simulink model "Hinf_BS_Comparison"  (R2026a)
settings: Solver=ode23tb  StopTime=175  FixedStep=0.0001  MaxStep=0.02  RelTol=1e-9  AbsTol=1e-12
PostLoadFcn:
  | init_comparison(bdroot);
InitFcn:
  | init_comparison(bdroot);
model workspace (MAT data in the model file):
  A = [-4.33427458178e-18 -1739.27628419 -1.9879507565e-12 -947.702562069 9.25490783271 -3.87188490855e-14 40.5994463199 -1.82279284791e-15 1.34368571874e-07 -8.90717137351e-10 -711.607566004 -711.607566004 ... (196 elements, 14x14)]
  B = [-1.75563782385e-19 2.23785567073e-19 -10165.2431057 -49.2726170531 5.13589910552 -5.90943945895 6.81435391425 45.4160051294 1073741824 17236611.4468 7.60467680903e-16 -1.03174259462e-14 ... (14 elements, 14x1)]
  C = [-313107.329042 -2686499.93691 37750.0108104 101565.096764 -37.2177294622 -2820.69827595 3048.09156473 3382.76066655 -2.10142044744 -107.98720369 -2843187.08558 -2796371.67099 ... (14 elements, 1x14)]
  D = 0
  a1 = 3
  a2 = 3
  a3 = 3
  a4 = 3
  b = -100
  k1 = 9.81
  k1_0 = 9.81
  k1_3 = 7.3575
  k2 = 0.555555555556
  k2_0 = 1.11111111111
  k2_3 = 6.66666666667
  k3 = 2.9
  k3_0 = 2
  k3_3 = 7.93333333333
  k4 = 1.8
  k4_0 = 0.9
  k4_3 = 0.45
  k5 = 0.620689655172
  k5_0 = 0.45
  k5_3 = 0.0567226890756
  r_test = [0 0.02 0.04 0.06 0.08 0.1 0.12 0.14 0.16 0.18 0.2 0.22 ... (17570 elements, 8785x2)]
  w = 500
(part 2 of 2)

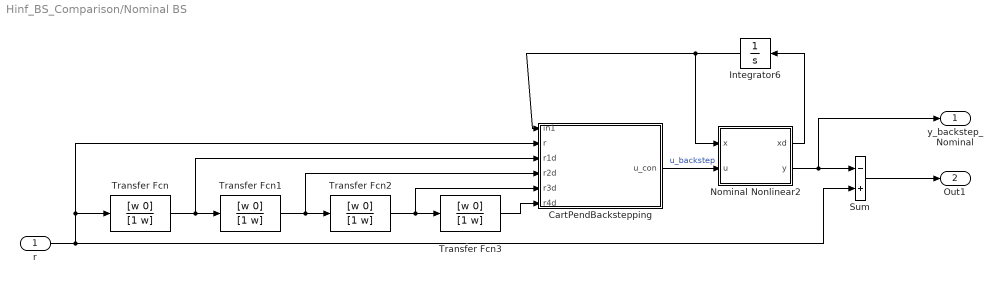
== system Hinf_BS_Comparison/Nominal BS ==
  r : Inport
  CartPendBackstepping : MATLAB Function  TreatAsAtomicUnit=on
  Integrator6 : Integrator  InitialCondition=zeros(4, 1)
  Nominal Nonlinear2 : MATLAB Function  TreatAsAtomicUnit=on
  Sum : Sum  Inputs=-+
  Transfer Fcn{,1..3} (4 alike) : TransferFcn  Numerator=[w 0]  Denominator=[1 w]
  y_backstep_Nominal : Outport
  Out1 : Outport  Port=2
  wires:
  Sum/1 -> Out1/1
  Nominal Nonlinear2/2(y) -> y_backstep_Nominal/1, Sum/1
  Transfer Fcn3/1 -> CartPendBackstepping/6(r4d)
  Transfer Fcn1/1 -> Transfer Fcn2/1, CartPendBackstepping/4(r2d)
  Nominal Nonlinear2/1(xd) -> Integrator6/1
  Transfer Fcn/1 -> Transfer Fcn1/1, CartPendBackstepping/3(r1d)
  Transfer Fcn2/1 -> Transfer Fcn3/1, CartPendBackstepping/5(r3d)
  Integrator6/1 -> CartPendBackstepping/1(in1), Nominal Nonlinear2/1(x)
  CartPendBackstepping/1(u_con) -> Nominal Nonlinear2/2(u)  "u_backstep"
  r/1 -> CartPendBackstepping/2(r), Transfer Fcn/1, Sum/2

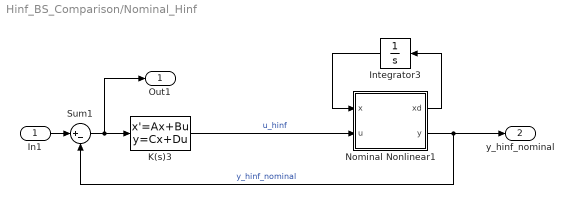
== system Hinf_BS_Comparison/Nominal_Hinf ==
  In1 : Inport
  Integrator3 : Integrator  InitialCondition=zeros(4, 1)
  K(s)3 : StateSpace  A=A  B=B  C=C  D=D  InitialCondition=0
  Nominal Nonlinear1 : MATLAB Function  TreatAsAtomicUnit=on
  Sum1 : Sum  Inputs=|+-
  Out1 : Outport
  y_hinf_nominal : Outport  Port=2
  wires:
  In1/1 -> Sum1/1
  Integrator3/1 -> Nominal Nonlinear1/1(x)
  Nominal Nonlinear1/2(y) -> y_hinf_nominal/1, Sum1/2  "y_hinf_nominal"
  K(s)3/1 -> Nominal Nonlinear1/2(u)  "u_hinf"
  Nominal Nonlinear1/1(xd) -> Integrator3/1
  Sum1/1 -> Out1/1, K(s)3/1

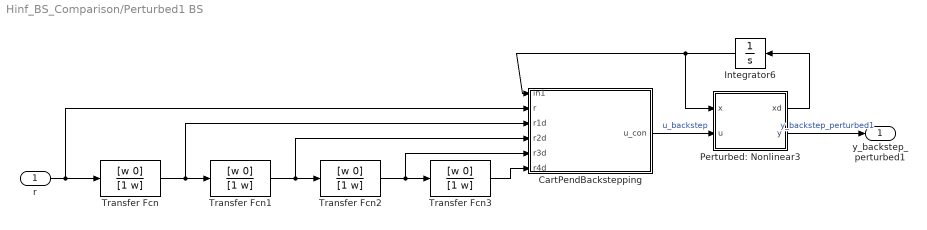
== system Hinf_BS_Comparison/Perturbed1 BS ==
  r : Inport
  CartPendBackstepping : MATLAB Function  TreatAsAtomicUnit=on
  Integrator6 : Integrator  InitialCondition=zeros(4, 1)
  Perturbed: Nonlinear3 : MATLAB Function  TreatAsAtomicUnit=on
  Transfer Fcn{,1..3} (4 alike) : TransferFcn  Numerator=[w 0]  Denominator=[1 w]
  y_backstep_perturbed1 : Outport
  wires:
  Integrator6/1 -> CartPendBackstepping/1(in1), Perturbed: Nonlinear3/1(x)
  Transfer Fcn3/1 -> CartPendBackstepping/6(r4d)
  Transfer Fcn2/1 -> Transfer Fcn3/1, CartPendBackstepping/5(r3d)
  Perturbed: Nonlinear3/1(xd) -> Integrator6/1
  CartPendBackstepping/1(u_con) -> Perturbed: Nonlinear3/2(u)  "u_backstep"
  Transfer Fcn/1 -> Transfer Fcn1/1, CartPendBackstepping/3(r1d)
  Transfer Fcn1/1 -> Transfer Fcn2/1, CartPendBackstepping/4(r2d)
  Perturbed: Nonlinear3/2(y) -> y_backstep_perturbed1/1  "y_backstep_perturbed1"
  r/1 -> CartPendBackstepping/2(r), Transfer Fcn/1

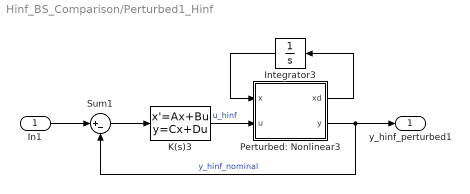
== system Hinf_BS_Comparison/Perturbed1_Hinf ==
  In1 : Inport
  Integrator3 : Integrator  InitialCondition=zeros(4, 1)
  K(s)3 : StateSpace  A=A  B=B  C=C  D=D  InitialCondition=0
  Perturbed: Nonlinear3 : MATLAB Function  TreatAsAtomicUnit=on
  Sum1 : Sum  Inputs=|+-
  y_hinf_perturbed1 : Outport
  wires:
  Integrator3/1 -> Perturbed: Nonlinear3/1(x)
  Perturbed: Nonlinear3/2(y) -> y_hinf_perturbed1/1, Sum1/2  "y_hinf_nominal"
  K(s)3/1 -> Perturbed: Nonlinear3/2(u)  "u_hinf"
  Perturbed: Nonlinear3/1(xd) -> Integrator3/1
  Sum1/1 -> K(s)3/1
  In1/1 -> Sum1/1

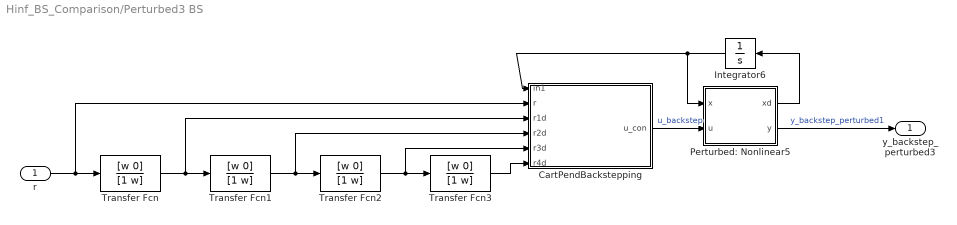
== system Hinf_BS_Comparison/Perturbed3 BS ==
  r : Inport
  CartPendBackstepping : MATLAB Function  TreatAsAtomicUnit=on
  Integrator6 : Integrator  InitialCondition=zeros(4, 1)
  Perturbed: Nonlinear5 : MATLAB Function  TreatAsAtomicUnit=on
  Transfer Fcn{,1..3} (4 alike) : TransferFcn  Numerator=[w 0]  Denominator=[1 w]
  y_backstep_perturbed3 : Outport
  wires:
  Integrator6/1 -> Perturbed: Nonlinear5/1(x), CartPendBackstepping/1(in1)
  Transfer Fcn3/1 -> CartPendBackstepping/6(r4d)
  Transfer Fcn2/1 -> Transfer Fcn3/1, CartPendBackstepping/5(r3d)
  Perturbed: Nonlinear5/1(xd) -> Integrator6/1
  CartPendBackstepping/1(u_con) -> Perturbed: Nonlinear5/2(u)  "u_backstep"
  Transfer Fcn/1 -> Transfer Fcn1/1, CartPendBackstepping/3(r1d)
  Transfer Fcn1/1 -> Transfer Fcn2/1, CartPendBackstepping/4(r2d)
  Perturbed: Nonlinear5/2(y) -> y_backstep_perturbed3/1  "y_backstep_perturbed1"
  r/1 -> Transfer Fcn/1, CartPendBackstepping/2(r)

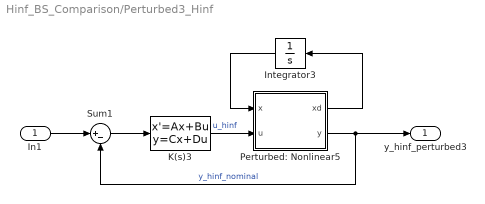
== system Hinf_BS_Comparison/Perturbed3_Hinf ==
  In1 : Inport
  Integrator3 : Integrator  InitialCondition=zeros(4, 1)
  K(s)3 : StateSpace  A=A  B=B  C=C  D=D  InitialCondition=0
  Perturbed: Nonlinear5 : MATLAB Function  TreatAsAtomicUnit=on
  Sum1 : Sum  Inputs=|+-
  y_hinf_perturbed3 : Outport
  wires:
  Integrator3/1 -> Perturbed: Nonlinear5/1(x)
  Perturbed: Nonlinear5/2(y) -> y_hinf_perturbed3/1, Sum1/2  "y_hinf_nominal"
  K(s)3/1 -> Perturbed: Nonlinear5/2(u)  "u_hinf"
  Perturbed: Nonlinear5/1(xd) -> Integrator3/1
  Sum1/1 -> K(s)3/1
  In1/1 -> Sum1/1

== matlab function Hinf_BS_Comparison/Perturbed3_Hinf/Perturbed: Nonlinear5 ==
  data: x input; u input; xd output; k1_3 parameter; k2_3 parameter; k3_3 parameter; k4_3 parameter; k5_3 parameter; b parameter; y output
function [xd, y] = cart_pend(x, u, k1_3, k2_3, k3_3, k4_3, k5_3, b)
xd = [x(2);
      -b^2*x(1) + 2*b*x(2) + b^2*u;
      x(4);
      (-k1_3*sin(x(3)) - k2_3*x(4) - cos(x(3))/k3_3 .* (x(1) + k4_3*sin(x(3)).*x(4).^2))./(1 - k5_3*cos(x(3)).^2)];
y = x(3);

== matlab function Hinf_BS_Comparison/Perturbed3 BS/CartPendBackstepping ==
  data: in1 input; u_con output; r input; r1d input; r2d input; r3d input; r4d input; a1 parameter; a2 parameter; a3 parameter; a4 parameter
function u_con = CartPendBackstepping(in1,r,r1d,r2d,r3d,r4d,a1, a2, a3, a4)
%#codegen


p1 = in1(1,:);
p2 = in1(2,:);
x1 = in1(3,:);
x2 = in1(4,:);
t2 = cos(x1);
t3 = sin(x1);
t4 = a1.*a2;
t5 = x1.*2.0;
t6 = x2.^2;
t7 = x2.^3;
t16 = -x1;
t17 = -x2;
t24 = x2.*(1.0e+1./9.0);
t8 = cos(t5);
t9 = t2.^2;
t10 = t2.^3;
t12 = t2.^5;
t14 = sin(t5);
t15 = t3.^3;
t18 = p1.*t3.*5.0e+1;
t19 = t2.*9.81e+2;
t22 = (p1.*t2)./2.0;
t28 = t3.*(9.81e+2./1.0e+2);
t34 = t2.*t3.*t6.*(9.0./2.0e+1);
t11 = t9.^2;
t13 = t9.^3;
t20 = t8.*9.0;
t21 = t9.*9.0;
t23 = -t18;
t25 = t8.*8.1e+1;
t26 = t14.*x2.*1.62e+2;
t27 = t8.*(9.0./2.0);
t32 = t6.*t14.*(9.0./4.0e+1);
t42 = t22+t24+t28+t34;
t29 = t20-3.1e+1;
t30 = t21-2.0e+1;
t31 = t26+4.0e+2;
t33 = t25-2.79e+2;
t37 = t27-3.1e+1./2.0;
t43 = t22+t24+t28+t32;
t35 = 1.0./t30;
t38 = 1.0./t33;
t39 = 1.0./t37;
t36 = t35.^2;
t40 = t31.*t38;
t41 = a1+a2+t40;
et1 = a1.*3.6e+5+a3.*3.6e+5-t2.*3.1392e+6-t6.*9.0e+5+t10.*5.2974e+6-a1.*t2.*3.5316e+5-a2.*t2.*3.5316e+5-a3.*t2.*3.5316e+5+a1.*t6.*1.62e+5+a3.*t4.*3.6e+5+a2.*t6.*1.62e+5+a3.*t6.*1.62e+5-a1.*t9.*4.86e+5-a1.*t10.*1.430298e+6+a1.*t11.*2.187e+5-a2.*t10.*1.430298e+6-a3.*t9.*4.86e+5+a1.*t12.*7.15149e+5-a3.*t10.*1.430298e+6-a1.*t13.*3.2805e+4;
et2 = a2.*t12.*7.15149e+5+a3.*t11.*2.187e+5+a3.*t12.*7.15149e+5-a3.*t13.*3.2805e+4-p1.*t3.*4.7e+5+p2.*t3.*1.8e+5+p1.*t15.*2.7e+5+t6.*t9.*5.85e+5+t6.*t11.*8.1e+5-t7.*t14.*4.05e+4+t3.*x2.*7.663572e+6-t14.*x2.*4.0e+5-t15.*x2.*1.0488852e+7+a1.*p1.*t3.*1.8e+5+a2.*p1.*t3.*1.8e+5+a3.*p1.*t3.*1.8e+5-a1.*t6.*t9.*3.24e+5-a3.*t4.*t9.*4.86e+5-a2.*t6.*t9.*3.24e+5+a1.*t6.*t11.*1.12995e+5;
et3 = a3.*t4.*t11.*2.187e+5-a3.*t6.*t9.*3.24e+5+a2.*t6.*t11.*1.12995e+5-a3.*t4.*t13.*3.2805e+4+a3.*t6.*t11.*1.12995e+5+a1.*t14.*x2.*1.8e+5+a2.*t14.*x2.*1.8e+5+a3.*t14.*x2.*1.8e+5-p2.*t3.*t11.*3.645e+4-p1.*t2.*x2.*6.3e+5+p1.*t10.*x2.*7.533e+5+p1.*t12.*x2.*1.0935e+5+t3.*t7.*t10.*6.7797e+5+t3.*t11.*x2.*2.145447e+6-a1.*p1.*t3.*t11.*3.645e+4-a2.*p1.*t3.*t11.*3.645e+4-a3.*p1.*t3.*t11.*3.645e+4-a1.*t3.*t10.*x2.*1.62e+5;
et4 = a2.*t3.*t10.*x2.*-1.62e+5-a3.*t3.*t10.*x2.*1.62e+5;
et5 = r4d+r1d.*(a1+a3+a3.*t4)+r3d.*(a1+a2+a3)+a4.*(r1d+r3d+t17+a1.*(r+t16)+t17.*(t4+(t19+t23+t6.*t8.*4.5e+1)./(t8.*(4.5e+1./2.0)-1.55e+2./2.0)+t14.*t39.^2.*t43.*1.8e+2+1.0)+r1d.*(t4+1.0)+a3.*(r+r2d+t16+a1.*r1d+a1.*t17+a2.*(r1d+t17+a1.*r+a1.*t16)-(t3.*8.829e+3+x2.*1.0e+3+p1.*t2.*4.5e+2+t6.*t14.*(4.05e+2./2.0))./(t8.*(4.05e+2./2.0)-6.975e+2))+r2d.*(a1+a2)-p2.*t2.*t39.*1.0e+1-t39.*t41.*t43.*2.0e+1)+r2d.*(t4+a1.*a3+a2.*a3+2.0)+t2.*t35.*(p1.*1.0e+5+p2.*2.0e+3);
et6 = (t35.^3.*x2.*(et1+et2+et3+et4))./4.5e+1-t35.*t42.*(t4+a3.*t41-(t6.*4.5e+1+t18-t19-t6.*t9.*9.0e+1)./(t9.*4.5e+1-1.0e+2)+1.0./t29.^2.*x2.*(t14.*8.0e+2+x2.*3.24e+2-t8.*x2.*1.116e+3)+(t41.*(t14.*x2.*(9.0./2.0e+1)+1.0e+1./9.0).*4.0e+1)./t29+t2.*t3.*t36.*t42.*7.2e+2+2.0).*2.0e+1-p2.*t36.*(t2.*2.0e+2-a1.*t2.*1.8e+2-a2.*t2.*1.8e+2-a3.*t2.*1.8e+2+a1.*t10.*8.1e+1+a2.*t10.*8.1e+1+a3.*t10.*8.1e+1+t3.*x2.*1.8e+2+t3.*t9.*x2.*2.43e+2).*(1.0e+1./9.0);
u_con = ((et5+et6).*(t9.*(9.0./2.0e+1)-1.0))./(t2.*5.0e+3);

% Complete the final recursion: dot(z3) = -a4*z3 - z2.
a_nom = (-9.81*sin(x1)-x2/0.9-0.5*p1*cos(x1) ...
    -0.45*cos(x1)*sin(x1)*x2.^2)./(1-0.45*cos(x1).^2);
b_nom = -0.5*cos(x1)./(1-0.45*cos(x1).^2);
z2 = r2d-a_nom+(a1+a2).*(r1d-x2)+(a1.*a2+1).*(r-x1);
u_con = u_con + z2./(1.0e4*b_nom);
end

== matlab function Hinf_BS_Comparison/Perturbed3 BS/Perturbed: Nonlinear5 ==
  data: x input; u input; xd output; k1_3 parameter; k2_3 parameter; k3_3 parameter; k4_3 parameter; k5_3 parameter; b parameter; y output
function [xd, y] = cart_pend(x, u, k1_3, k2_3, k3_3, k4_3, k5_3, b)
xd = [x(2);
      -b^2*x(1) + 2*b*x(2) + b^2*u;
      x(4);
      (-k1_3*sin(x(3)) - k2_3*x(4) - cos(x(3))/k3_3 .* (x(1) + k4_3*sin(x(3)).*x(4).^2))./(1 - k5_3*cos(x(3)).^2)];
y = x(3);

== matlab function Hinf_BS_Comparison/Nominal_Hinf/Nominal Nonlinear1 ==
  data: x input; u input; xd output; k1_0 parameter; k2_0 parameter; k3_0 parameter; k4_0 parameter; k5_0 parameter; b parameter; y output
function [xd, y] = cart_pend(x, u, k1_0, k2_0, k3_0, k4_0, k5_0, b)

xd = [x(2);
      -b^2*x(1) + 2*b*x(2) + b^2*u;
      x(4);
      (-k1_0*sin(x(3)) - k2_0*x(4) - cos(x(3))/k3_0 .* (x(1) + k4_0*sin(x(3)).*x(4).^2))./(1 - k5_0*cos(x(3)).^2)];

y = x(3);

== matlab function Hinf_BS_Comparison/Nominal BS/CartPendBackstepping ==
  data: in1 input; u_con output; r input; r1d input; r2d input; r3d input; r4d input; a1 parameter; a2 parameter; a3 parameter; a4 parameter
function u_con = CartPendBackstepping(in1,r,r1d,r2d,r3d,r4d,a1, a2, a3, a4)
%#codegen


p1 = in1(1,:);
p2 = in1(2,:);
x1 = in1(3,:);
x2 = in1(4,:);
t2 = cos(x1);
t3 = sin(x1);
t4 = a1.*a2;
t5 = x1.*2.0;
t6 = x2.^2;
t7 = x2.^3;
t16 = -x1;
t17 = -x2;
t24 = x2.*(1.0e+1./9.0);
t8 = cos(t5);
t9 = t2.^2;
t10 = t2.^3;
t12 = t2.^5;
t14 = sin(t5);
t15 = t3.^3;
t18 = p1.*t3.*5.0e+1;
t19 = t2.*9.81e+2;
t22 = (p1.*t2)./2.0;
t28 = t3.*(9.81e+2./1.0e+2);
t34 = t2.*t3.*t6.*(9.0./2.0e+1);
t11 = t9.^2;
t13 = t9.^3;
t20 = t8.*9.0;
t21 = t9.*9.0;
t23 = -t18;
t25 = t8.*8.1e+1;
t26 = t14.*x2.*1.62e+2;
t27 = t8.*(9.0./2.0);
t32 = t6.*t14.*(9.0./4.0e+1);
t42 = t22+t24+t28+t34;
t29 = t20-3.1e+1;
t30 = t21-2.0e+1;
t31 = t26+4.0e+2;
t33 = t25-2.79e+2;
t37 = t27-3.1e+1./2.0;
t43 = t22+t24+t28+t32;
t35 = 1.0./t30;
t38 = 1.0./t33;
t39 = 1.0./t37;
t36 = t35.^2;
t40 = t31.*t38;
t41 = a1+a2+t40;
et1 = a1.*3.6e+5+a3.*3.6e+5-t2.*3.1392e+6-t6.*9.0e+5+t10.*5.2974e+6-a1.*t2.*3.5316e+5-a2.*t2.*3.5316e+5-a3.*t2.*3.5316e+5+a1.*t6.*1.62e+5+a3.*t4.*3.6e+5+a2.*t6.*1.62e+5+a3.*t6.*1.62e+5-a1.*t9.*4.86e+5-a1.*t10.*1.430298e+6+a1.*t11.*2.187e+5-a2.*t10.*1.430298e+6-a3.*t9.*4.86e+5+a1.*t12.*7.15149e+5-a3.*t10.*1.430298e+6-a1.*t13.*3.2805e+4;
et2 = a2.*t12.*7.15149e+5+a3.*t11.*2.187e+5+a3.*t12.*7.15149e+5-a3.*t13.*3.2805e+4-p1.*t3.*4.7e+5+p2.*t3.*1.8e+5+p1.*t15.*2.7e+5+t6.*t9.*5.85e+5+t6.*t11.*8.1e+5-t7.*t14.*4.05e+4+t3.*x2.*7.663572e+6-t14.*x2.*4.0e+5-t15.*x2.*1.0488852e+7+a1.*p1.*t3.*1.8e+5+a2.*p1.*t3.*1.8e+5+a3.*p1.*t3.*1.8e+5-a1.*t6.*t9.*3.24e+5-a3.*t4.*t9.*4.86e+5-a2.*t6.*t9.*3.24e+5+a1.*t6.*t11.*1.12995e+5;
et3 = a3.*t4.*t11.*2.187e+5-a3.*t6.*t9.*3.24e+5+a2.*t6.*t11.*1.12995e+5-a3.*t4.*t13.*3.2805e+4+a3.*t6.*t11.*1.12995e+5+a1.*t14.*x2.*1.8e+5+a2.*t14.*x2.*1.8e+5+a3.*t14.*x2.*1.8e+5-p2.*t3.*t11.*3.645e+4-p1.*t2.*x2.*6.3e+5+p1.*t10.*x2.*7.533e+5+p1.*t12.*x2.*1.0935e+5+t3.*t7.*t10.*6.7797e+5+t3.*t11.*x2.*2.145447e+6-a1.*p1.*t3.*t11.*3.645e+4-a2.*p1.*t3.*t11.*3.645e+4-a3.*p1.*t3.*t11.*3.645e+4-a1.*t3.*t10.*x2.*1.62e+5;
et4 = a2.*t3.*t10.*x2.*-1.62e+5-a3.*t3.*t10.*x2.*1.62e+5;
et5 = r4d+r1d.*(a1+a3+a3.*t4)+r3d.*(a1+a2+a3)+a4.*(r1d+r3d+t17+a1.*(r+t16)+t17.*(t4+(t19+t23+t6.*t8.*4.5e+1)./(t8.*(4.5e+1./2.0)-1.55e+2./2.0)+t14.*t39.^2.*t43.*1.8e+2+1.0)+r1d.*(t4+1.0)+a3.*(r+r2d+t16+a1.*r1d+a1.*t17+a2.*(r1d+t17+a1.*r+a1.*t16)-(t3.*8.829e+3+x2.*1.0e+3+p1.*t2.*4.5e+2+t6.*t14.*(4.05e+2./2.0))./(t8.*(4.05e+2./2.0)-6.975e+2))+r2d.*(a1+a2)-p2.*t2.*t39.*1.0e+1-t39.*t41.*t43.*2.0e+1)+r2d.*(t4+a1.*a3+a2.*a3+2.0)+t2.*t35.*(p1.*1.0e+5+p2.*2.0e+3);
et6 = (t35.^3.*x2.*(et1+et2+et3+et4))./4.5e+1-t35.*t42.*(t4+a3.*t41-(t6.*4.5e+1+t18-t19-t6.*t9.*9.0e+1)./(t9.*4.5e+1-1.0e+2)+1.0./t29.^2.*x2.*(t14.*8.0e+2+x2.*3.24e+2-t8.*x2.*1.116e+3)+(t41.*(t14.*x2.*(9.0./2.0e+1)+1.0e+1./9.0).*4.0e+1)./t29+t2.*t3.*t36.*t42.*7.2e+2+2.0).*2.0e+1-p2.*t36.*(t2.*2.0e+2-a1.*t2.*1.8e+2-a2.*t2.*1.8e+2-a3.*t2.*1.8e+2+a1.*t10.*8.1e+1+a2.*t10.*8.1e+1+a3.*t10.*8.1e+1+t3.*x2.*1.8e+2+t3.*t9.*x2.*2.43e+2).*(1.0e+1./9.0);
u_con = ((et5+et6).*(t9.*(9.0./2.0e+1)-1.0))./(t2.*5.0e+3);

% Complete the final recursion: dot(z3) = -a4*z3 - z2.
a_nom = (-9.81*sin(x1)-x2/0.9-0.5*p1*cos(x1) ...
    -0.45*cos(x1)*sin(x1)*x2.^2)./(1-0.45*cos(x1).^2);
b_nom = -0.5*cos(x1)./(1-0.45*cos(x1).^2);
z2 = r2d-a_nom+(a1+a2).*(r1d-x2)+(a1.*a2+1).*(r-x1);
u_con = u_con + z2./(1.0e4*b_nom);
end

== matlab function Hinf_BS_Comparison/Nominal BS/Nominal Nonlinear2 ==
  data: x input; u input; xd output; k1_0 parameter; k2_0 parameter; k3_0 parameter; k4_0 parameter; k5_0 parameter; b parameter; y output
function [xd, y] = cart_pend(x, u, k1_0, k2_0, k3_0, k4_0, k5_0, b)

xd = [x(2);
      -b^2*x(1) + 2*b*x(2) + b^2*u;
      x(4);
      (-k1_0*sin(x(3)) - k2_0*x(4) - cos(x(3))/k3_0 .* (x(1) + k4_0*sin(x(3)).*x(4).^2))./(1 - k5_0*cos(x(3)).^2)];

y = x(3);

== matlab function Hinf_BS_Comparison/Perturbed1 BS/CartPendBackstepping ==
  data: in1 input; u_con output; r input; r1d input; r2d input; r3d input; r4d input; a1 parameter; a2 parameter; a3 parameter; a4 parameter
function u_con = CartPendBackstepping(in1,r,r1d,r2d,r3d,r4d,a1, a2, a3, a4)
%#codegen


p1 = in1(1,:);
p2 = in1(2,:);
x1 = in1(3,:);
x2 = in1(4,:);
t2 = cos(x1);
t3 = sin(x1);
t4 = a1.*a2;
t5 = x1.*2.0;
t6 = x2.^2;
t7 = x2.^3;
t16 = -x1;
t17 = -x2;
t24 = x2.*(1.0e+1./9.0);
t8 = cos(t5);
t9 = t2.^2;
t10 = t2.^3;
t12 = t2.^5;
t14 = sin(t5);
t15 = t3.^3;
t18 = p1.*t3.*5.0e+1;
t19 = t2.*9.81e+2;
t22 = (p1.*t2)./2.0;
t28 = t3.*(9.81e+2./1.0e+2);
t34 = t2.*t3.*t6.*(9.0./2.0e+1);
t11 = t9.^2;
t13 = t9.^3;
t20 = t8.*9.0;
t21 = t9.*9.0;
t23 = -t18;
t25 = t8.*8.1e+1;
t26 = t14.*x2.*1.62e+2;
t27 = t8.*(9.0./2.0);
t32 = t6.*t14.*(9.0./4.0e+1);
t42 = t22+t24+t28+t34;
t29 = t20-3.1e+1;
t30 = t21-2.0e+1;
t31 = t26+4.0e+2;
t33 = t25-2.79e+2;
t37 = t27-3.1e+1./2.0;
t43 = t22+t24+t28+t32;
t35 = 1.0./t30;
t38 = 1.0./t33;
t39 = 1.0./t37;
t36 = t35.^2;
t40 = t31.*t38;
t41 = a1+a2+t40;
et1 = a1.*3.6e+5+a3.*3.6e+5-t2.*3.1392e+6-t6.*9.0e+5+t10.*5.2974e+6-a1.*t2.*3.5316e+5-a2.*t2.*3.5316e+5-a3.*t2.*3.5316e+5+a1.*t6.*1.62e+5+a3.*t4.*3.6e+5+a2.*t6.*1.62e+5+a3.*t6.*1.62e+5-a1.*t9.*4.86e+5-a1.*t10.*1.430298e+6+a1.*t11.*2.187e+5-a2.*t10.*1.430298e+6-a3.*t9.*4.86e+5+a1.*t12.*7.15149e+5-a3.*t10.*1.430298e+6-a1.*t13.*3.2805e+4;
et2 = a2.*t12.*7.15149e+5+a3.*t11.*2.187e+5+a3.*t12.*7.15149e+5-a3.*t13.*3.2805e+4-p1.*t3.*4.7e+5+p2.*t3.*1.8e+5+p1.*t15.*2.7e+5+t6.*t9.*5.85e+5+t6.*t11.*8.1e+5-t7.*t14.*4.05e+4+t3.*x2.*7.663572e+6-t14.*x2.*4.0e+5-t15.*x2.*1.0488852e+7+a1.*p1.*t3.*1.8e+5+a2.*p1.*t3.*1.8e+5+a3.*p1.*t3.*1.8e+5-a1.*t6.*t9.*3.24e+5-a3.*t4.*t9.*4.86e+5-a2.*t6.*t9.*3.24e+5+a1.*t6.*t11.*1.12995e+5;
et3 = a3.*t4.*t11.*2.187e+5-a3.*t6.*t9.*3.24e+5+a2.*t6.*t11.*1.12995e+5-a3.*t4.*t13.*3.2805e+4+a3.*t6.*t11.*1.12995e+5+a1.*t14.*x2.*1.8e+5+a2.*t14.*x2.*1.8e+5+a3.*t14.*x2.*1.8e+5-p2.*t3.*t11.*3.645e+4-p1.*t2.*x2.*6.3e+5+p1.*t10.*x2.*7.533e+5+p1.*t12.*x2.*1.0935e+5+t3.*t7.*t10.*6.7797e+5+t3.*t11.*x2.*2.145447e+6-a1.*p1.*t3.*t11.*3.645e+4-a2.*p1.*t3.*t11.*3.645e+4-a3.*p1.*t3.*t11.*3.645e+4-a1.*t3.*t10.*x2.*1.62e+5;
et4 = a2.*t3.*t10.*x2.*-1.62e+5-a3.*t3.*t10.*x2.*1.62e+5;
et5 = r4d+r1d.*(a1+a3+a3.*t4)+r3d.*(a1+a2+a3)+a4.*(r1d+r3d+t17+a1.*(r+t16)+t17.*(t4+(t19+t23+t6.*t8.*4.5e+1)./(t8.*(4.5e+1./2.0)-1.55e+2./2.0)+t14.*t39.^2.*t43.*1.8e+2+1.0)+r1d.*(t4+1.0)+a3.*(r+r2d+t16+a1.*r1d+a1.*t17+a2.*(r1d+t17+a1.*r+a1.*t16)-(t3.*8.829e+3+x2.*1.0e+3+p1.*t2.*4.5e+2+t6.*t14.*(4.05e+2./2.0))./(t8.*(4.05e+2./2.0)-6.975e+2))+r2d.*(a1+a2)-p2.*t2.*t39.*1.0e+1-t39.*t41.*t43.*2.0e+1)+r2d.*(t4+a1.*a3+a2.*a3+2.0)+t2.*t35.*(p1.*1.0e+5+p2.*2.0e+3);
et6 = (t35.^3.*x2.*(et1+et2+et3+et4))./4.5e+1-t35.*t42.*(t4+a3.*t41-(t6.*4.5e+1+t18-t19-t6.*t9.*9.0e+1)./(t9.*4.5e+1-1.0e+2)+1.0./t29.^2.*x2.*(t14.*8.0e+2+x2.*3.24e+2-t8.*x2.*1.116e+3)+(t41.*(t14.*x2.*(9.0./2.0e+1)+1.0e+1./9.0).*4.0e+1)./t29+t2.*t3.*t36.*t42.*7.2e+2+2.0).*2.0e+1-p2.*t36.*(t2.*2.0e+2-a1.*t2.*1.8e+2-a2.*t2.*1.8e+2-a3.*t2.*1.8e+2+a1.*t10.*8.1e+1+a2.*t10.*8.1e+1+a3.*t10.*8.1e+1+t3.*x2.*1.8e+2+t3.*t9.*x2.*2.43e+2).*(1.0e+1./9.0);
u_con = ((et5+et6).*(t9.*(9.0./2.0e+1)-1.0))./(t2.*5.0e+3);

% Complete the final recursion: dot(z3) = -a4*z3 - z2.
a_nom = (-9.81*sin(x1)-x2/0.9-0.5*p1*cos(x1) ...
    -0.45*cos(x1)*sin(x1)*x2.^2)./(1-0.45*cos(x1).^2);
b_nom = -0.5*cos(x1)./(1-0.45*cos(x1).^2);
z2 = r2d-a_nom+(a1+a2).*(r1d-x2)+(a1.*a2+1).*(r-x1);
u_con = u_con + z2./(1.0e4*b_nom);
end

== matlab function Hinf_BS_Comparison/Perturbed1 BS/Perturbed: Nonlinear3 ==
  data: x input; u input; xd output; k1 parameter; k2 parameter; k3 parameter; k4 parameter; k5 parameter; b parameter; y output
function [xd, y] = cart_pend(x, u, k1, k2, k3, k4, k5, b)

xd = [x(2);
      -b^2*x(1) + 2*b*x(2) + b^2*u;
      x(4);
      (-k1*sin(x(3)) - k2*x(4) - cos(x(3))/k3 .* (x(1) + k4*sin(x(3)).*x(4).^2))./(1 - k5*cos(x(3)).^2)];

y = x(3);

== matlab function Hinf_BS_Comparison/Perturbed1_Hinf/Perturbed: Nonlinear3 ==
  data: x input; u input; xd output; k1 parameter; k2 parameter; k3 parameter; k4 parameter; k5 parameter; b parameter; y output
function [xd, y] = cart_pend(x, u, k1, k2, k3, k4, k5, b)

xd = [x(2);
      -b^2*x(1) + 2*b*x(2) + b^2*u;
      x(4);
      (-k1*sin(x(3)) - k2*x(4) - cos(x(3))/k3 .* (x(1) + k4*sin(x(3)).*x(4).^2))./(1 - k5*cos(x(3)).^2)];

y = x(3);
